simulink model "Vehicle_system_Adaptive_MPC"  (R2024b)
settings: configuration reference "vehicle_config" (kept outside this file)
settings Model: DataDictionary=sim_data_vehicle.sldd  SILPILSystemUnderTest=refmodels  Creator=tshintai  LastModifiedBy=tshintai
settings ConfigSetRef: SourceName=vehicle_config

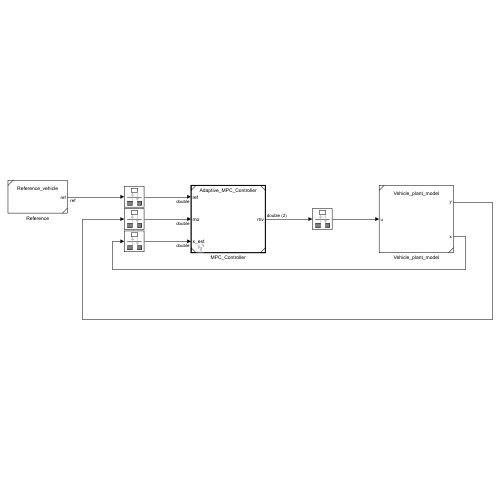
[thumbnail: Simulink's stored preview of the top-level diagram]
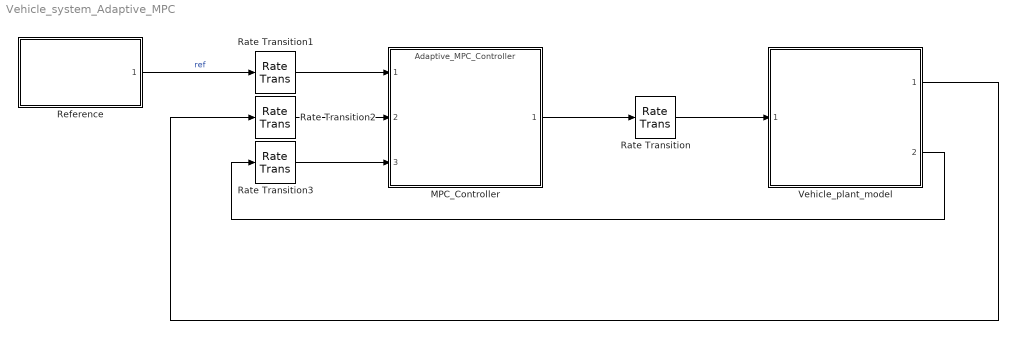
== system Vehicle_system_Adaptive_MPC ==
  MPC_Controller : ModelReference  ModelNameDialog=Adaptive_MPC_Controller.slx  SimulationMode=Normal  ModelReferenceVersion=8.0
  Rate Transition{,1..3} (4 alike) : RateTransition  OutPortSampleTime=TimeStep
  Reference : Subsystem  ReferencedSubsystem=Reference_vehicle
  Vehicle_plant_model : Subsystem  ReferencedSubsystem=Vehicle_plant_model
  wires:
  Reference/1 -> Rate Transition1/1  "ref"
  Rate Transition/1 -> Vehicle_plant_model/1
  Vehicle_plant_model/1 -> Rate Transition2/1
  Rate Transition1/1 -> MPC_Controller/1
  Rate Transition2/1 -> MPC_Controller/2
  Vehicle_plant_model/2 -> Rate Transition3/1
  Rate Transition3/1 -> MPC_Controller/3
  MPC_Controller/1 -> Rate Transition/1
